simulink model "week2_problem1"  (R2019b)
settings: Solver=VariableStepAuto  StartTime=0.0  StopTime=5000  RelTol=1e-3
settings Model: Creator=Shreyas  LastModifiedBy=Shreyas

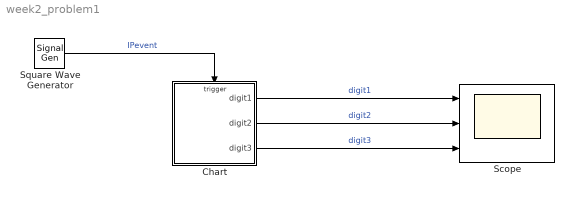
== system week2_problem1 ==
  Chart : Stateflow chart  BlockKeywords=__PRM__SERIALIZED__DATA__:Stateflow Chart,Stateflow Diagram  TreatAsAtomicUnit=on
  Scope : Scope  NumInputPorts=3
  Square Wave Generator : SignalGenerator  WaveForm=square  Units=rad/sec
  wires:
  Square Wave Generator/1 -> Chart/Trigger  "IPevent"
  Chart/1(digit1) -> Scope/1  "digit1"
  Chart/2(digit2) -> Scope/2  "digit2"
  Chart/3(digit3) -> Scope/3  "digit3"

== stateflow chart week2_problem1/Chart ==
  state States_Counter
    state D2 [parallel]
      settings: executionOrder=1
      state one
        en: digit2 = 1;
      state two
        en: digit2 = 2;
      state zero
        en: digit2 = 0;
      state three
        en:digit2=3;
      state four
        en:digit2=4;
      States_Counter.D2.zero -> States_Counter.D2.one : inc2
      States_Counter.D2.one -> States_Counter.D2.two : inc2
      (default) -> States_Counter.D2.zero
      States_Counter.D2.four -> States_Counter.D2.zero : inc2{D3.inc3;}
      States_Counter.D2.two -> States_Counter.D2.three : inc2
      States_Counter.D2.three -> States_Counter.D2.four : inc2
    state D3 [parallel]
      settings: executionOrder=2
      state one
        en: digit3 = 1;
      state two
        en: digit3 = 2;
      state zero
        en: digit3 = 0;
      state three
        en:digit3=3;
      state four
        en:digit3=4;
      States_Counter.D3.one -> States_Counter.D3.two : inc3
      States_Counter.D3.zero -> States_Counter.D3.one : inc3
      (default) -> States_Counter.D3.zero
      States_Counter.D3.two -> States_Counter.D3.three : inc3
      States_Counter.D3.four -> States_Counter.D3.zero : inc3
      States_Counter.D3.three -> States_Counter.D3.four : inc3
    state D1 [parallel]
      settings: executionOrder=3
      state one
        en: digit1 = 1;
      state two
        en: digit1 = 2;
      state zero
        en: digit1 = 0;
      state three
        en:digit1=3;
      state four
        en:digit1=4;
      States_Counter.D1.zero -> States_Counter.D1.one : IPevent
      States_Counter.D1.one -> States_Counter.D1.two : IPevent
      (default) -> States_Counter.D1.zero
      States_Counter.D1.four -> States_Counter.D1.zero : IPevent{D2.inc2;}
      States_Counter.D1.two -> States_Counter.D1.three : IPevent
      States_Counter.D1.three -> States_Counter.D1.four : IPevent
  data: digit1 output; digit2 output; digit3 output
  events: inc2 local FUNCTION_CALL_EVENT; inc3 local FUNCTION_CALL_EVENT; IPevent input EITHER_EDGE_EVENT
